simulink library "old_courseFollow_cl"  (R2018b)
settings: Solver=VariableStepAuto  StartTime=0.0  StopTime=10.0  RelTol=1e-3
undefined symbols (not defined in the file or in its folder): a
libraries: $bdroot x6, dspindex x2, vectorNormalizer_ul x2, schmehlTangentRotation_ul x1, angleBtw2DVecs_ul x1, tangVecToPath x1
settings Model: Creator=James Reed  LastModifiedBy=James Reed

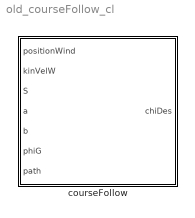
== system old_courseFollow_cl ==
  courseFollow : Subsystem

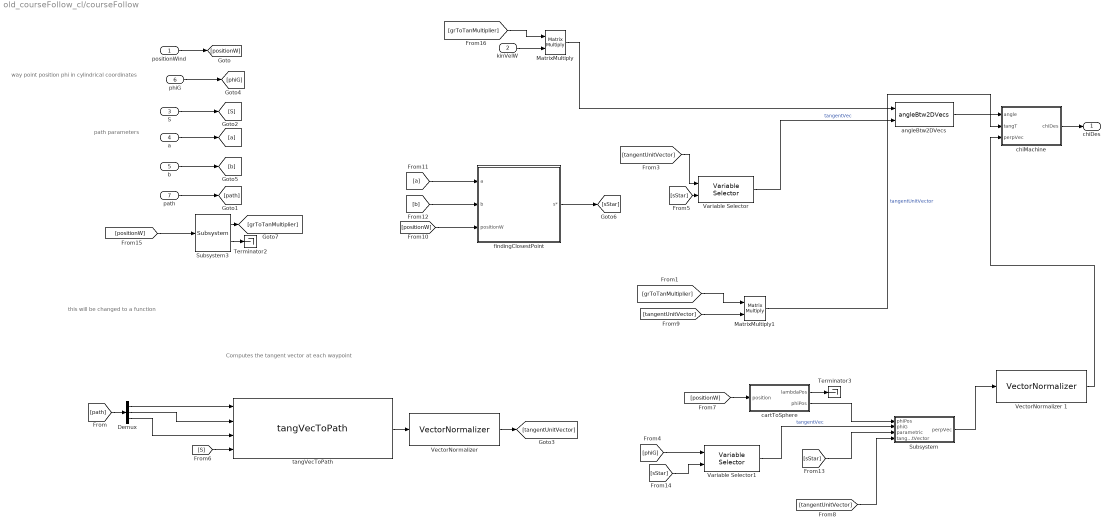
== system old_courseFollow_cl/courseFollow ==
  note: this will be changed to a function
  note: way point position phi in cylindrical coordinates
  note: path parameters
  note: Computes the tangent vector at each waypoint
  "positionWind " : Inport
  kinVelW : Inport  Port=2
  S : Inport  Port=3
  a : Inport  Port=4
  "b " : Inport  Port=5
  phiG : Inport  Port=6
  path : Inport  Port=7
  Demux : Demux  Outputs=3
  MatrixMultiply : Product  Multiplication=Matrix(*)
  MatrixMultiply1 : Product  Multiplication=Matrix(*)
  Subsystem : Subsystem
  Subsystem3 : schmehlTangentRotation_ul/Subsystem  SystemSampleTime=-1
  Terminator2 : Terminator
  Terminator3 : Terminator
  Variable Selector : dspindex/Variable Selector  NumInputs=1  rowsOrCols=Columns  IdxMode=Variable  Elements=[1 3]  ZerOneIdxMode=One-based  errmode=Clip Index  FillMode=on  FillValues=0
  Variable Selector1 : dspindex/Variable Selector  NumInputs=1  rowsOrCols=Columns  IdxMode=Variable  Elements=[1 3]  ZerOneIdxMode=One-based  errmode=Clip Index  FillMode=on  FillValues=0
  "VectorNormalizer " : vectorNormalizer_ul/VectorNormalizer   SystemSampleTime=-1
  VectorNormalizer 1 : vectorNormalizer_ul/VectorNormalizer   SystemSampleTime=-1
  angleBtw2DVecs : angleBtw2DVecs_ul/angleBtw2DVecs  SystemSampleTime=-1
  cartToSphere : Subsystem
  chiMachine : Subsystem
  findingClosestPoint : Subsystem
  tangVecToPath : tangVecToPath/tangVecToPath  SystemSampleTime=-1
  "chiDes " : Outport
  wires:
  tangVecToPath/1 -> "VectorNormalizer "/1
  MatrixMultiply1/1 -> chiMachine/2(tangT)  "tangentUnitVector"
  Variable Selector/1 -> angleBtw2DVecs/2  "tangentVec"
  kinVelW/1 -> MatrixMultiply/2
  MatrixMultiply/1 -> angleBtw2DVecs/1
  "positionWind "/1 -> [positionW]
  [grToTanMultiplier] -> MatrixMultiply1/1
  Demux/2 -> tangVecToPath/2
  Demux/3 -> tangVecToPath/3
  angleBtw2DVecs/1 -> chiMachine/1("angle ")
  chiMachine/1("chiDes ") -> "chiDes "/1
  S/1 -> [S]
  [S] -> tangVecToPath/4
  [positionW] -> cartToSphere/1(position)
  "VectorNormalizer "/1 -> [tangentUnitVector]
  [tangentUnitVector] -> Subsystem/4("tangentUnitVector ")
  [tangentUnitVector] -> MatrixMultiply1/2
  [positionW] -> findingClosestPoint/3(positionW)
  a/1 -> [a]
  "b "/1 -> [b]
  [a] -> findingClosestPoint/1(a)
  [b] -> findingClosestPoint/2(b)
  [sStar] -> Subsystem/3("parametric ")
  path/1 -> [path]
  [path] -> Demux/1
  Demux/1 -> tangVecToPath/1
  [tangentUnitVector] -> Variable Selector/1
  findingClosestPoint/1(s*) -> [sStar]
  phiG/1 -> [phiG]
  [phiG] -> Variable Selector1/1
  [sStar] -> Variable Selector/2
  [sStar] -> Variable Selector1/2
  Subsystem/1(perpVec) -> VectorNormalizer 1/1
  VectorNormalizer 1/1 -> chiMachine/3("perpVec ")
  [positionW] -> Subsystem3/1
  Subsystem3/2 -> Terminator2/1
  Subsystem3/1 -> [grToTanMultiplier]
  [grToTanMultiplier] -> MatrixMultiply/1
  cartToSphere/1(lambdaPos) -> Terminator3/1
  cartToSphere/2(phiPos) -> Subsystem/1(phiPos)
  Variable Selector1/1 -> Subsystem/2(phiG)  "tangentVec"

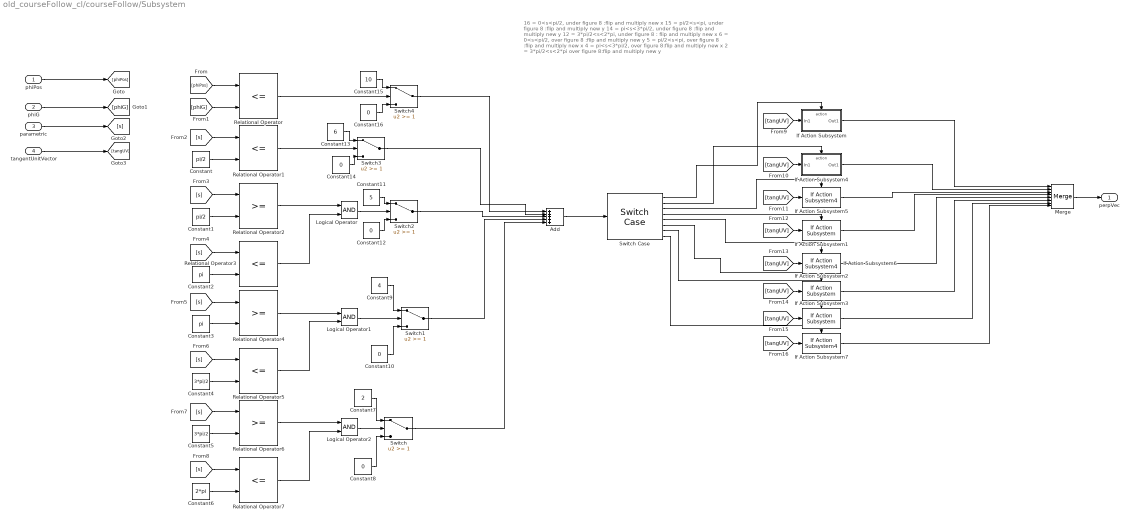
== system old_courseFollow_cl/courseFollow/Subsystem ==
  note: 16 = 0<s<pi/2, under figure 8 :flip and multiply new x
      | 15 = pi/2<s<pi, under figure 8  :flip and multiply new y
      | 14 = pi<s<3*pi/2, under figure 8 :flip and multiply new y
      | 12 = 3*pi/2<s<2*pi, under figure 8 : flip and multiply new x
      | 6 = 0<s<pi/2, over figure 8 :flip and multiply new y
      | 5 = pi/2<s<pi, over figure 8 :flip and multiply new x
      | 4 = pi<s<3*pi/2, over figure 8:flip and multiply new x
      | 2 = 3*pi/2<s<2*pi over figure 8:flip and multiply new y
  phiPos : Inport
  phiG : Inport  Port=2
  "parametric " : Inport  Port=3
  "tangentUnitVector " : Inport  Port=4
  Add : Sum  Inputs=+++++
  Constant : Constant  Value=pi/2
  Constant1 : Constant  Value=pi/2
  Constant{8,10,12,14,16} (5 alike) : Constant  Value=0
  Constant11 : Constant  Value=5
  Constant13 : Constant  Value=6
  Constant15 : Constant  Value=10
  Constant2 : Constant  Value=pi
  Constant3 : Constant  Value=pi
  Constant4 : Constant  Value=3*pi/2
  Constant5 : Constant  Value=3*pi/2
  Constant6 : Constant  Value=2*pi
  Constant7 : Constant  Value=2
  Constant9 : Constant  Value=4
  If Action Subsystem : Subsystem  TreatAsAtomicUnit=on
  If Action Subsystem1 : $bdroot/courseFollow/Subsystem/If Action Subsystem  SystemSampleTime=-1
  If Action Subsystem2 : $bdroot/courseFollow/Subsystem/If Action Subsystem  SystemSampleTime=-1
  If Action Subsystem3 : $bdroot/courseFollow/Subsystem/If Action Subsystem  SystemSampleTime=-1
  If Action Subsystem4 : Subsystem  TreatAsAtomicUnit=on
  If Action Subsystem5 : $bdroot/courseFollow/Subsystem/If Action Subsystem4  SystemSampleTime=-1
  If Action Subsystem6 : $bdroot/courseFollow/Subsystem/If Action Subsystem4  SystemSampleTime=-1
  If Action Subsystem7 : $bdroot/courseFollow/Subsystem/If Action Subsystem4  SystemSampleTime=-1
  Logical Operator : Logic  AllPortsSameDT=off  OutDataTypeStr=boolean
  Logical Operator1 : Logic  AllPortsSameDT=off  OutDataTypeStr=boolean
  Logical Operator2 : Logic  AllPortsSameDT=off  OutDataTypeStr=boolean
  Merge : Merge  Inputs=8
  Relational Operator{,1,3,5,7} (5 alike) : RelationalOperator  Operator=<=  OutDataTypeStr=boolean  RndMeth=Simplest
  Relational Operator2 : RelationalOperator  OutDataTypeStr=boolean  RndMeth=Simplest
  Relational Operator4 : RelationalOperator  OutDataTypeStr=boolean  RndMeth=Simplest
  Relational Operator6 : RelationalOperator  OutDataTypeStr=boolean  RndMeth=Simplest
  Switch{,1..4} (5 alike) : Switch  Threshold=1
  Switch Case : SwitchCase  CaseConditions={16,15,14,12,6,5,4,2}  ShowDefaultCase=off
  perpVec : Outport
  wires:
  phiPos/1 -> [phiPos]
  phiG/1 -> [phiG]
  Relational Operator/1 -> Switch4/2
  [phiPos] -> Relational Operator/1
  [phiG] -> Relational Operator/2
  "parametric "/1 -> [s]
  [s] -> Relational Operator1/1
  Constant/1 -> Relational Operator1/2
  [s] -> Relational Operator2/1
  Constant1/1 -> Relational Operator2/2
  Relational Operator2/1 -> Logical Operator/1
  [s] -> Relational Operator3/1
  Constant2/1 -> Relational Operator3/2
  Relational Operator3/1 -> Logical Operator/2
  Relational Operator4/1 -> Logical Operator1/1
  [s] -> Relational Operator4/1
  Constant4/1 -> Relational Operator5/2
  Constant3/1 -> Relational Operator4/2
  [s] -> Relational Operator5/1
  Relational Operator5/1 -> Logical Operator1/2
  Relational Operator6/1 -> Logical Operator2/1
  [s] -> Relational Operator6/1
  Constant6/1 -> Relational Operator7/2
  Constant5/1 -> Relational Operator6/2
  [s] -> Relational Operator7/1
  Relational Operator7/1 -> Logical Operator2/2
  Logical Operator2/1 -> Switch/2
  Constant7/1 -> Switch/1
  Constant8/1 -> Switch/3
  Logical Operator1/1 -> Switch1/2
  Constant9/1 -> Switch1/1
  Constant10/1 -> Switch1/3
  Logical Operator/1 -> Switch2/2
  Constant11/1 -> Switch2/1
  Constant12/1 -> Switch2/3
  Constant13/1 -> Switch3/1
  Constant14/1 -> Switch3/3
  Relational Operator1/1 -> Switch3/2
  Constant15/1 -> Switch4/1
  Constant16/1 -> Switch4/3
  Switch4/1 -> Add/1
  Switch3/1 -> Add/2
  Switch2/1 -> Add/3
  Switch1/1 -> Add/4
  Switch/1 -> Add/5
  Add/1 -> Switch Case/1
  Switch Case/1 -> If Action Subsystem/Action
  Switch Case/2 -> If Action Subsystem4/Action
  Switch Case/3 -> If Action Subsystem5/Action
  Switch Case/4 -> If Action Subsystem1/Action
  Switch Case/5 -> If Action Subsystem6/Action
  Switch Case/6 -> If Action Subsystem2/Action
  Switch Case/7 -> If Action Subsystem3/Action
  Switch Case/8 -> If Action Subsystem7/Action
  "tangentUnitVector "/1 -> [tangUV]
  [tangUV] -> If Action Subsystem/1(In1)
  [tangUV] -> If Action Subsystem4/1(In1)
  [tangUV] -> If Action Subsystem5/1
  [tangUV] -> If Action Subsystem1/1
  [tangUV] -> If Action Subsystem6/1
  [tangUV] -> If Action Subsystem2/1
  [tangUV] -> If Action Subsystem3/1
  [tangUV] -> If Action Subsystem7/1
  If Action Subsystem/1(Out1) -> Merge/1
  If Action Subsystem4/1(Out1) -> Merge/2
  If Action Subsystem5/1 -> Merge/3
  If Action Subsystem1/1 -> Merge/4
  If Action Subsystem6/1 -> Merge/5
  If Action Subsystem2/1 -> Merge/6
  If Action Subsystem3/1 -> Merge/7
  If Action Subsystem7/1 -> Merge/8
  Merge/1 -> perpVec/1

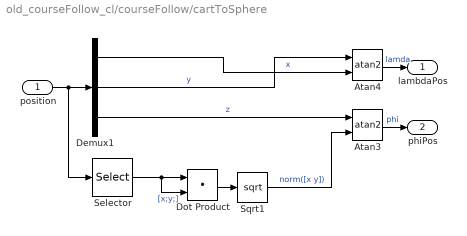
== system old_courseFollow_cl/courseFollow/cartToSphere ==
  position : Inport
  Atan3 : Trigonometry  Operator=atan2
  Atan4 : Trigonometry  Operator=atan2
  Demux1 : Demux  Outputs=3
  Dot Product : DotProduct  InputSameDT=on  OutDataTypeStr=Inherit: Inherit via internal rule
  Selector : Selector  InputPortWidth=3  IndexOptions=Index vector (dialog)  Indices=[1 2]  OutputSizes=1
  Sqrt1 : Sqrt  SaturateOnIntegerOverflow=on
  lambdaPos : Outport
  phiPos : Outport  Port=2
  wires:
  position/1 -> Demux1/1, Selector/1
  Dot Product/1 -> Sqrt1/1
  Demux1/3 -> Atan3/1  "z"
  Demux1/2 -> Atan4/1  "y"
  Demux1/1 -> Atan4/2  "x"
  Selector/1 -> Dot Product/1, Dot Product/2  "[x;y;]"
  Sqrt1/1 -> Atan3/2  "norm([x y])"
  Atan4/1 -> lambdaPos/1  "lamda"
  Atan3/1 -> phiPos/1  "phi"

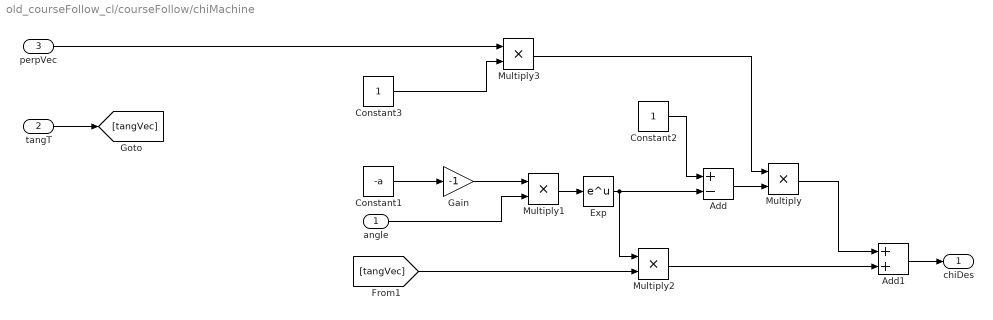
== system old_courseFollow_cl/courseFollow/chiMachine ==
  "angle " : Inport
  tangT : Inport  Port=2
  "perpVec " : Inport  Port=3
  Add : Sum  Inputs=+-
  Add1 : Sum
  Constant1 : Constant  Value=-a
  Constant2 : Constant
  Constant3 : Constant
  Exp : Math  SaturateOnIntegerOverflow=on
  Gain : Gain  Gain=-1
  Multiply{,1..3} (4 alike) : Product
  "chiDes " : Outport
  wires:
  tangT/1 -> [tangVec]
  Constant1/1 -> Gain/1
  Gain/1 -> Multiply1/1
  "angle "/1 -> Multiply1/2
  Multiply1/1 -> Exp/1
  Exp/1 -> Add/2, Multiply2/1
  Constant2/1 -> Add/1
  [tangVec] -> Multiply2/2
  Multiply3/1 -> Multiply/1
  Constant3/1 -> Multiply3/2
  Add/1 -> Multiply/2
  Multiply/1 -> Add1/1
  Multiply2/1 -> Add1/2
  Add1/1 -> "chiDes "/1
  "perpVec "/1 -> Multiply3/1

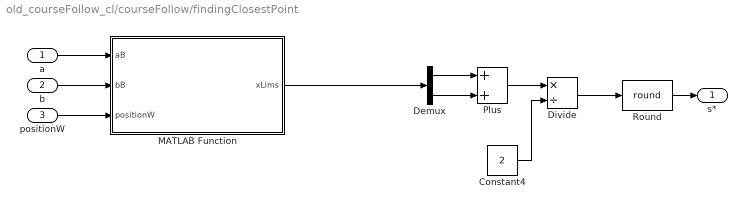
== system old_courseFollow_cl/courseFollow/findingClosestPoint ==
  a : Inport
  b : Inport  Port=2
  positionW : Inport  Port=3
  Constant4 : Constant  Value=2
  Demux : Demux  Outputs=2
  Divide : Product  Inputs=*/
  MATLAB Function : MATLAB Function  TreatAsAtomicUnit=on
  Plus : Sum
  Round : Rounding  Operator=round
  s* : Outport
  wires:
  MATLAB Function/1(xLims) -> Demux/1
  Demux/2 -> Plus/2
  Demux/1 -> Plus/1
  Plus/1 -> Divide/1
  Constant4/1 -> Divide/2
  Divide/1 -> Round/1
  Round/1 -> s*/1
  a/1 -> MATLAB Function/1(aB)
  b/1 -> MATLAB Function/2(bB)
  positionW/1 -> MATLAB Function/3(positionW)

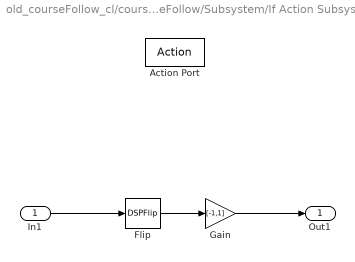
== system old_courseFollow_cl/courseFollow/Subsystem/If Action Subsystem ==
  In1 : Inport
  Action Port : ActionPort  ActionType=case
  Flip : DSPFlip
  Gain : Gain  Gain=[-1,1]
  Out1 : Outport
  wires:
  In1/1 -> Flip/1
  Flip/1 -> Gain/1
  Gain/1 -> Out1/1

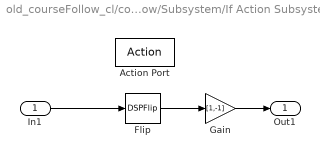
== system old_courseFollow_cl/courseFollow/Subsystem/If Action Subsystem4 ==
  In1 : Inport
  Action Port : ActionPort  ActionType=case
  Flip : DSPFlip
  Gain : Gain  Gain=[1,-1]
  Out1 : Outport
  wires:
  Flip/1 -> Gain/1
  In1/1 -> Flip/1
  Gain/1 -> Out1/1

== matlab function old_courseFollow_cl/courseFollow/findingClosestPoint/MATLAB Function ==
  data: aB input; xLims output; bB input; positionW input
function xLims  = fcn(aB,bB,positionW)

     centralAngle = @(s)(2.*asin(.5*(norm( [(cos(((aB.*sin(s))./(1 + ((aB/bB)^2).*(cos(s).^2)))).*cos(((((aB/bB)^2).*sin(s).*cos(s))./(1 + ((aB/bB)^2).*(cos(s).^2)))));
                        (sin(((aB.*sin(s))./(1 + ((aB/bB)^2).*(cos(s).^2)))).*cos(((((aB/bB)^2).*sin(s).*cos(s))./(1 + ((aB/bB)^2).*(cos(s).^2)))));
                        (sin(((((aB/bB)^2).*sin(s).*cos(s))./(1 + ((aB/bB)^2).*(cos(s).^2)))));]-positionW))));


   
s0 = 1; % Point to start searching from
stepSize  = 1; % Size of the jump to use between guesses
xLims = goldenSection(s0,stepSize,'FunctionHandle',centralAngle);
